simulink model "task2_att"  (R2024b)
settings: Solver=VariableStepAuto  StartTime=0.0  StopTime=10.0  RelTol=1e-3
values from neighbouring files (symbols this model uses):
  omegab_0 = [0 0 0]'    [MAIN.m]    (also in MAIN_exam_2025.m)
  q_0 = eul2quat([0, theta_cmd, 0 ]*degToRad,'ZYX')'    [MAIN.m]    (also in MAIN_exam_2025.m = eul2quat([0, 0, 0 ]*degToRad,'XYZ')')
  UAV = include_pack(UAV,pack,1)    [MAIN.m]
undefined symbols (not defined in the file or in its folder): ctrl
libraries: matrix_library x1
settings Model: Creator=invernizzi  LastModifiedBy=ggera

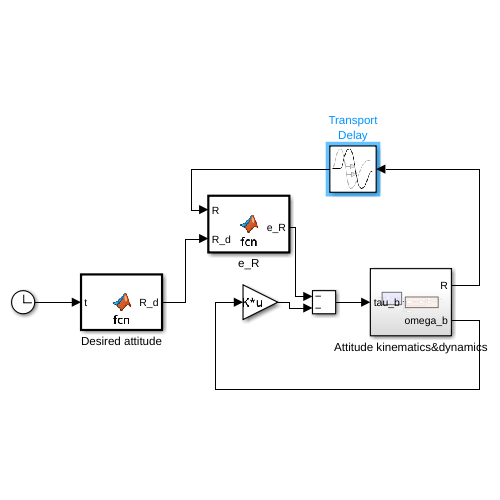
[thumbnail: Simulink's stored preview of the top-level diagram]
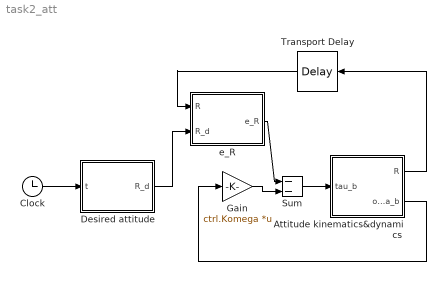
== system task2_att ==
  Attitude kinematics&dynamics : Subsystem
  Clock : Clock
  Desired attitude : MATLAB Function  TreatAsAtomicUnit=on
  Gain : Gain  Gain=ctrl.Komega  Multiplication=Matrix(K*u)
  Sum : Sum  Inputs=--
  Transport Delay : TransportDelay  DelayTime=0.01  InitialOutput=eye(3)
  e_R : MATLAB Function  TreatAsAtomicUnit=on
  wires:
  Sum/1 -> Attitude kinematics&dynamics/1(tau_b)
  Gain/1 -> Sum/2
  Attitude kinematics&dynamics/2(omega_b) -> Gain/1
  Clock/1 -> Desired attitude/1(t)
  Desired attitude/1(R_d) -> e_R/2(R_d)
  Attitude kinematics&dynamics/1(R) -> Transport Delay/1
  e_R/1(e_R) -> Sum/1
  Transport Delay/1 -> e_R/1(R)

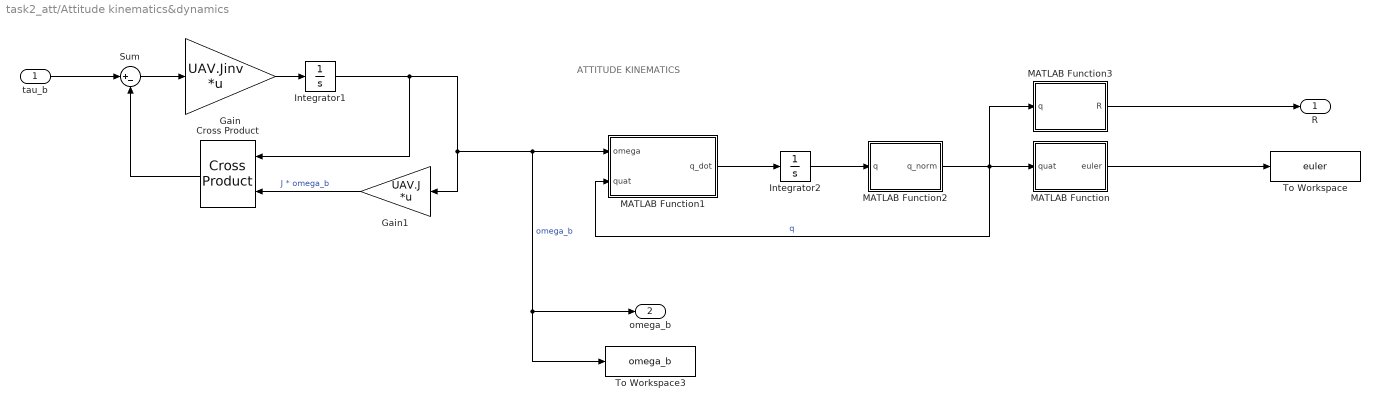
== system task2_att/Attitude kinematics&dynamics ==
  note: ATTITUDE KINEMATICS
  tau_b : Inport
  Cross Product : matrix_library/Cross Product
  Gain : Gain  Gain=UAV.Jinv  Multiplication=Matrix(K*u)
  Gain1 : Gain  Gain=UAV.J  Multiplication=Matrix(K*u)
  Integrator1 : Integrator  InitialCondition=omegab_0
  Integrator2 : Integrator  InitialCondition=q_0
  MATLAB Function : MATLAB Function  TreatAsAtomicUnit=on
  MATLAB Function1 : MATLAB Function  TreatAsAtomicUnit=on
  MATLAB Function2 : MATLAB Function  TreatAsAtomicUnit=on
  MATLAB Function3 : MATLAB Function  TreatAsAtomicUnit=on
  Sum : Sum  Inputs=|+-
  To Workspace : ToWorkspace  VariableName=euler  SaveFormat=Timeseries  SampleTime=-1
  To Workspace3 : ToWorkspace  VariableName=omega_b  SaveFormat=Timeseries  SampleTime=-1
  R : Outport
  omega_b : Outport  Port=2
  wires:
  MATLAB Function/1(euler) -> To Workspace/1
  Integrator1/1 -> Cross Product/1, omega_b/1, To Workspace3/1, MATLAB Function1/1(omega), Gain1/1  "omega_b"
  MATLAB Function2/1(q_norm) -> MATLAB Function3/1(q), MATLAB Function1/2(quat), MATLAB Function/1(quat)  "q"
  Integrator2/1 -> MATLAB Function2/1(q)
  MATLAB Function1/1(q_dot) -> Integrator2/1
  Sum/1 -> Gain/1
  Gain/1 -> Integrator1/1
  MATLAB Function3/1(R) -> R/1
  Gain1/1 -> Cross Product/2  "J * omega_b"
  tau_b/1 -> Sum/1
  Cross Product/1 -> Sum/2

== matlab function task2_att/Attitude kinematics&dynamics/MATLAB Function ==
  data: quat input; euler output
function euler = quatToEuler( quat )
%	Converts a quaternion vector to ZYX Euler angles (RPY)

euler = quat2eul(quat','ZYX');

end

== matlab function task2_att/Attitude kinematics&dynamics/MATLAB Function2 ==
  data: q input; q_norm output
function q_norm = quat_norm( q )

norm = sqrt( q(1)^2 + q(2)^2 + q(3)^2 + q(4)^2 );

q_norm = 1/norm * q;

== matlab function task2_att/Attitude kinematics&dynamics/MATLAB Function3 ==
  data: q input; R output
function R = fcn(q)

R = quat2rotm(q');

end

== matlab function task2_att/Desired attitude ==
  data: t input; R_d output; par parameter
function R_d = fcn(t,par)

R_d = eul2rotm(par.eul_d);

== matlab function task2_att/e_R ==
  data: R input; e_R output; R_d input; par parameter
function e_R = fcn(R,R_d,par)

k_R1 = par.k_R1;
k_R2 = par.k_R2;
k_R3 = par.k_R3;

e_1 = [1 0 0]';
e_2 = [0 1 0]';
e_3 = [0 0 1]';
R_e = R_d'*R; % transformation from body to desired frame coordinates

e_R = k_R1*cross(R_e'*e_1,e_1) + k_R2*cross(R_e'*e_2,e_2) + k_R3*cross(R_e'*e_3,e_3);

== matlab function task2_att/Attitude kinematics&dynamics/MATLAB Function1 ==
  data: omega input; quat input; q_dot output
 function q_dot = quat_kin(omega, quat)
%#codegen

eta = quat(1);
eps = quat(2:4);

W=[-eps';
   skew(eps) + eta*eye(3)];

q_dot = 0.5*W*omega;

end

function S=skew(s)
S=[0  -s(3)  s(2);
    s(3)   0 -s(1);
    -s(2)  s(1)  0];
end
